simulink model "GA_GearBox"  (R2020a)
settings: Solver=ode23t  StartTime=0.0  StopTime=1  FixedStep=Tsamp  RelTol=1e-3  AbsTol=1e-3  EnableMultiTasking=on
InitFcn:
  | Gear_parameters
StopFcn:
  | Gear_plot
values from neighbouring files (symbols this model uses):
  backlash1_bound = 0.3157*0.1    (= 0.03157)    [Gear_parameters.m]
  backlash2_bound = 0.3157*0.1    (= 0.03157)    [Gear_parameters.m]
  backlash3_bound = 0.2966*0.1    (= 0.02966)    [Gear_parameters.m]
  backlash4_bound = 0.3157*0.1    (= 0.03157)    [Gear_parameters.m]
undefined symbols (not defined in the file or in its folder): sigbuilder_block
libraries: fl_lib x28, nesl_utility x18, sdl_lib x4
Description:
  | Gear with Backlash
settings Model: FPTRunName=Active  ExtModeAutoUpdateStatusClock=off  Creator=MathWorks  LastModifiedBy=JSPark
settings SolverCC: AutoScaleAbsTol=off
settings DataIOCC: MaxDataPoints=10000  SaveFormat=Array  SignalLoggingSaveFormat=ModelDataLogs  SaveOutput=off  SignalLogging=off  DSMLogging=off  ReturnWorkspaceOutputs=off  SignalLoggingName=logsout_sdl_gear_backlash
settings OptimizationCC: ExpressionDepthLimit=2147483647  InitFltsAndDblsToZero=on  LifeSpan=inf
settings DebuggingCC: AlgebraicLoopMsg=none  SaveWithParameterizedLinksMsg=none  SignalResolutionControl=TryResolveAllWithWarning  MultiTaskDSMMsg=warning  MultiTaskCondExecSysMsg=none  SigSpecEnsureSampleTimeMsg=none  StateNameClashWarn=warning  PregeneratedLibrarySubsystemCodeDiagnostic=none  SFUnexpectedBacktrackingDiag=warning  SFNoUnconditionalDefaultTransitionDiag=warning  SFExecutionAtInitializationDiag=none  ArithmeticOperatorsInVariantConditions=warning
settings HardwareCC: ProdBitPerPointer=32  ProdBitPerSizeT=32  ProdBitPerPtrDiffT=32  ProdLargestAtomicFloat=None  ProdIntDivRoundTo=Undefined  ProdEndianess=Unspecified  ProdWordSize=32  ProdHWDeviceType=32-bit Generic  TargetBitPerPointer=64  TargetBitPerSizeT=64  TargetBitPerPtrDiffT=64  TargetLongLongMode=on  TargetIntDivRoundTo=Zero  TargetEndianess=LittleEndian  TargetWordSize=64  TargetHWDeviceType=MATLAB Host  ProdEqTarget=off
settings ModelReferenceCC: PropagateSignalLabelsOutOfModel=off
settings SFSimCC: SimUseLocalCustomCode=off  CustomCodeUndefinedFunction=UseInterfaceOnly
settings RTWCC: Description=Generic Real-Time Target  RTWUseLocalCustomCode=off
settings CodeAppCC: StateflowObjectComments=on
settings GRTTargetCC: TargetLangStandard=C89/C90 (ANSI)  CombineOutputUpdateFcns=off  GRTInterface=on
settings ConfigComp: CovMetricSettings=dw  CovHtmlReporting=on  CovSaveCumulativeToWorkspaceVar=on  CovSaveSingleToWorkspaceVar=on  CovShowResultsExplorer=off  CovExternalEMLEnable=off
settings SimscapeCC: SimscapeLogType=all  SimscapeLogSimulationStatistics=on  SimscapeLogName=simlog_sdl_gear_backlash  SimscapeLogLimitData=off  SimscapeLogDataHistory=15000

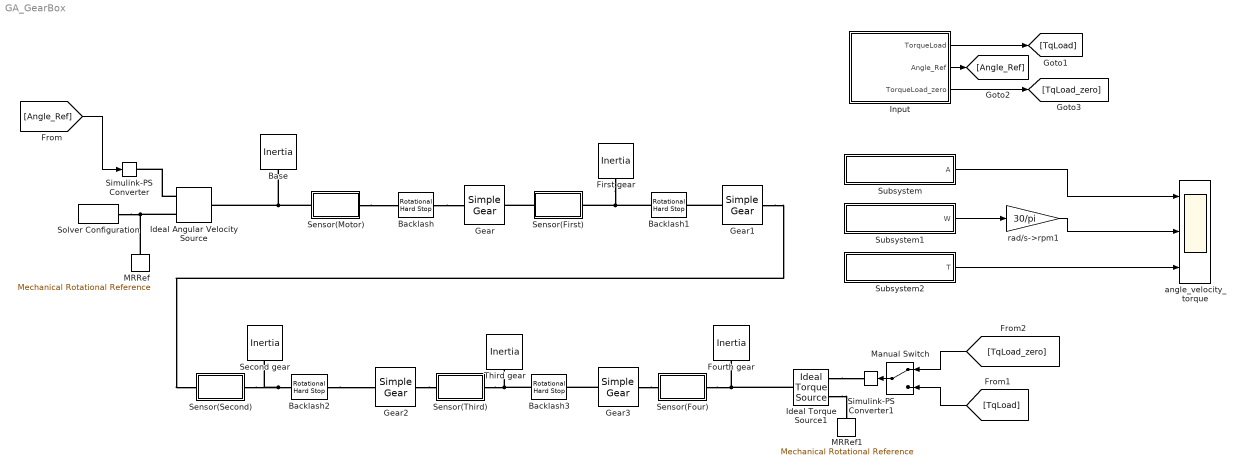
== system GA_GearBox ==
  Backlash : fl_lib/Mechanical/Rotational Elements/Rotational Hard Stop  upper_bnd=backlash1_bound deg  lower_bnd=-backlash1_bound deg  stiff_up=backlash1_stiffness N*m/rad  stiff_low=backlash1_stiffness N*m/rad  D_up=backlash1_damping N*m/(rad/s)  D_low=backlash1_damping N*m/(rad/s)  model=simscape.enum.hardstop.smooth  transition=backlash1_bound*0.1 deg  w_specify=off  w_priority=None  w=0 rad/s  w_nominal_specify=off  w_nominal_unit=rad/s  w_nominal_value=1  t_specify=off  t_priority=None  t=0 N*m  t_nominal_specify=off  t_nominal_unit=N*m  t_nominal_value=1  phi_specify=on  phi_priority=High  phi=0 rad  phi_nominal_specify=off  phi_nominal_unit=rad  phi_nominal_value=1
      settings: SourceProductBaseCode=SS
  Backlash1 : fl_lib/Mechanical/Rotational Elements/Rotational Hard Stop  upper_bnd=backlash2_bound deg  lower_bnd=-backlash2_bound deg  stiff_up=backlash2_stiffness N*m/rad  stiff_low=backlash2_stiffness N*m/rad  D_up=backlash2_damping N*m/(rad/s)  D_low=backlash2_damping N*m/(rad/s)  model=simscape.enum.hardstop.smooth  transition=backlash2_bound*0.1 deg  w_specify=off  w_priority=None  w=0 rad/s  w_nominal_specify=off  w_nominal_unit=rad/s  w_nominal_value=1  t_specify=off  t_priority=None  t=0 N*m  t_nominal_specify=off  t_nominal_unit=N*m  t_nominal_value=1  phi_specify=on  phi_priority=High  phi=0 rad  phi_nominal_specify=off  phi_nominal_unit=rad  phi_nominal_value=1
      settings: SourceProductBaseCode=SS
  Backlash2 : fl_lib/Mechanical/Rotational Elements/Rotational Hard Stop  upper_bnd=backlash3_bound deg  lower_bnd=-backlash3_bound deg  stiff_up=backlash3_stiffness N*m/rad  stiff_low=backlash3_stiffness N*m/rad  D_up=backlash3_damping N*m/(rad/s)  D_low=backlash3_damping N*m/(rad/s)  model=simscape.enum.hardstop.smooth  transition=backlash3_bound*0.1 deg  w_specify=off  w_priority=None  w=0 rad/s  w_nominal_specify=off  w_nominal_unit=rad/s  w_nominal_value=1  t_specify=off  t_priority=None  t=0 N*m  t_nominal_specify=off  t_nominal_unit=N*m  t_nominal_value=1  phi_specify=on  phi_priority=High  phi=0 rad  phi_nominal_specify=off  phi_nominal_unit=rad  phi_nominal_value=1
      settings: SourceProductBaseCode=SS
  Backlash3 : fl_lib/Mechanical/Rotational Elements/Rotational Hard Stop  upper_bnd=backlash4_bound deg  lower_bnd=-backlash4_bound deg  stiff_up=backlash4_stiffness N*m/rad  stiff_low=backlash4_stiffness N*m/rad  D_up=backlash4_damping N*m/(rad/s)  D_low=backlash4_damping N*m/(rad/s)  model=simscape.enum.hardstop.smooth  transition=backlash4_bound*0.1 deg  w_specify=off  w_priority=None  w=0 rad/s  w_nominal_specify=off  w_nominal_unit=rad/s  w_nominal_value=1  t_specify=off  t_priority=None  t=0 N*m  t_nominal_specify=off  t_nominal_unit=N*m  t_nominal_value=1  phi_specify=on  phi_priority=High  phi=0 rad  phi_nominal_specify=off  phi_nominal_unit=rad  phi_nominal_value=1
      settings: SourceProductBaseCode=SS
  Base : fl_lib/Mechanical/Rotational Elements/Inertia  inertia=Jm kg*m^2  w_specify=on  w_priority=High  w=0 rad/s  w_nominal_specify=off  w_nominal_unit=rad/s  w_nominal_value=1  t_specify=off  t_priority=None  t=0 N*m  t_nominal_specify=off  t_nominal_unit=N*m  t_nominal_value=1
  First gear : fl_lib/Mechanical/Rotational Elements/Inertia  inertia=gear_inertia1 kg*m^2  w_specify=on  w_priority=High  w=0 rad/s  w_nominal_specify=off  w_nominal_unit=rad/s  w_nominal_value=1  t_specify=off  t_priority=None  t=0 N*m  t_nominal_specify=off  t_nominal_unit=N*m  t_nominal_value=1
  Fourth gear : fl_lib/Mechanical/Rotational Elements/Inertia  inertia=gear_inertia4 kg*m^2  w_specify=on  w_priority=High  w=0 rad/s  w_nominal_specify=off  w_nominal_unit=rad/s  w_nominal_value=1  t_specify=off  t_priority=None  t=0 N*m  t_nominal_specify=off  t_nominal_unit=N*m  t_nominal_value=1
  Gear : sdl_lib/Gears/Simple Gear  ratio=gear_ratio1  rotation_direction=1  friction_model=sdl.enum.gear_efficiencies_load.off  T_noload=0.1 N*m  T_nom=5 N*m  efficiency_nom=0.8  efficiency=0.8  mu_visc=[ 0 0 ] N*m/(rad/s)  w_thr=0.01 rad/s  pwr_thr=0.001 W  enable_faults=simscape.enum.onoff.off  efficiency_fault=0.05  external_fault=simscape.enum.onoff.off  temporal_fault=simscape.enum.onoff.off  fault_time=5 s  fault_angles=pi / 12 rad  report_fault=1  temperature_TLU=[ 280 300 320 ] K  load_TLU=[ 1 5 10 ] N*m  efficiency_TLU=[ 0.95 0.9 0.85 ]  efficiency_TLU2=[ 0.85 0.8 0.75; 0.95 0.9 0.85; 0.85 0.8 0.7 ]  thermal_mass=50 J/K  T_init=300 K
  Gear1 : sdl_lib/Gears/Simple Gear  ratio=gear_ratio2  rotation_direction=1  friction_model=sdl.enum.gear_efficiencies_load.off  T_noload=0.1 N*m  T_nom=5 N*m  efficiency_nom=0.8  efficiency=0.8  mu_visc=[ 0 0 ] N*m/(rad/s)  w_thr=0.01 rad/s  pwr_thr=0.001 W  enable_faults=simscape.enum.onoff.off  efficiency_fault=0.05  external_fault=simscape.enum.onoff.off  temporal_fault=simscape.enum.onoff.off  fault_time=5 s  fault_angles=pi / 12 rad  report_fault=1  temperature_TLU=[ 280 300 320 ] K  load_TLU=[ 1 5 10 ] N*m  efficiency_TLU=[ 0.95 0.9 0.85 ]  efficiency_TLU2=[ 0.85 0.8 0.75; 0.95 0.9 0.85; 0.85 0.8 0.7 ]  thermal_mass=50 J/K  T_init=300 K
  Gear2 : sdl_lib/Gears/Simple Gear  ratio=gear_ratio3  rotation_direction=1  friction_model=sdl.enum.gear_efficiencies_load.off  T_noload=0.1 N*m  T_nom=5 N*m  efficiency_nom=0.8  efficiency=0.8  mu_visc=[ 0 0 ] N*m/(rad/s)  w_thr=0.01 rad/s  pwr_thr=0.001 W  enable_faults=simscape.enum.onoff.off  efficiency_fault=0.05  external_fault=simscape.enum.onoff.off  temporal_fault=simscape.enum.onoff.off  fault_time=5 s  fault_angles=pi / 12 rad  report_fault=1  temperature_TLU=[ 280 300 320 ] K  load_TLU=[ 1 5 10 ] N*m  efficiency_TLU=[ 0.95 0.9 0.85 ]  efficiency_TLU2=[ 0.85 0.8 0.75; 0.95 0.9 0.85; 0.85 0.8 0.7 ]  thermal_mass=50 J/K  T_init=300 K
  Gear3 : sdl_lib/Gears/Simple Gear  ratio=gear_ratio4  rotation_direction=1  friction_model=sdl.enum.gear_efficiencies_load.off  T_noload=0.1 N*m  T_nom=5 N*m  efficiency_nom=0.8  efficiency=0.8  mu_visc=[ 0 0 ] N*m/(rad/s)  w_thr=0.01 rad/s  pwr_thr=0.001 W  enable_faults=simscape.enum.onoff.off  efficiency_fault=0.05  external_fault=simscape.enum.onoff.off  temporal_fault=simscape.enum.onoff.off  fault_time=5 s  fault_angles=pi / 12 rad  report_fault=1  temperature_TLU=[ 280 300 320 ] K  load_TLU=[ 1 5 10 ] N*m  efficiency_TLU=[ 0.95 0.9 0.85 ]  efficiency_TLU2=[ 0.85 0.8 0.75; 0.95 0.9 0.85; 0.85 0.8 0.7 ]  thermal_mass=50 J/K  T_init=300 K
  Ideal Angular Velocity Source : fl_lib/Mechanical/Mechanical Sources/Ideal Angular Velocity Source
  Ideal Torque Source1 : fl_lib/Mechanical/Mechanical Sources/Ideal Torque Source
  Input : Subsystem  Tag=STV Subsys  LoadFcn=sigbuilder_block('load');  StartFcn=sigbuilder_block('start');  StopFcn=sigbuilder_block('stop');  ClipboardFcn=sigbuilder_block('clipboard');  mask(Sigbuilder block){tuvar=[0:10]}
      mask help: Simulink:masks:SigbuilderBlock_MD
      mask init:
      | if ~strcmp(get_param(bdroot(gcbh),'SimulationStatus'),'stopped') tuvar = sigbuilder_block('maskInit'); end
      settings: CopyFcn=sigbuilder_block('copy');  DeleteFcn=sigbuilder_block('delete');  ModelCloseFcn=sigbuilder_block('modelClose');  PreSaveFcn=sigbuilder_block('preSave');  PauseFcn=sigbuilder_block('pause');  ContinueFcn=sigbuilder_block('continue');  NameChangeFcn=sigbuilder_block('namechange');  OpenFcn=sigbuilder_block('open',[661.5 288 949.5 474.75 ]);  CloseFcn=sigbuilder_block('close');
      mask Display: plot(0, 0, 100, 100,[2, 2, 32, 32, 2], [68, 8, 8, 68, 68],[32, 2], [38, 38], [32, 19, 2],[53, 60, 44], [32, 17, 17, 2],[16, 16, 31, 31]);txt = getActiveGroup(gcbh);text(2, 100, txt,'verticalAlignment', 'top');
  MRRef : fl_lib/Mechanical/Rotational Elements/Mechanical Rotational Reference
  MRRef1 : fl_lib/Mechanical/Rotational Elements/Mechanical Rotational Reference
  Manual Switch : ManualSwitch
  Second gear : fl_lib/Mechanical/Rotational Elements/Inertia  inertia=gear_inertia2 kg*m^2  w_specify=on  w_priority=High  w=0 rad/s  w_nominal_specify=off  w_nominal_unit=rad/s  w_nominal_value=1  t_specify=off  t_priority=None  t=0 N*m  t_nominal_specify=off  t_nominal_unit=N*m  t_nominal_value=1
  Sensor(First) : Subsystem
  Sensor(Four) : Subsystem
  Sensor(Motor) : Subsystem
  Sensor(Second) : Subsystem
  Sensor(Third) : Subsystem
  Simulink-PS Converter : nesl_utility/Simulink-PS Converter  PhysicalDomain=network_engine_domain  SubClassName=ps_input  LeftPortType=input  RightPortType=output  PseudoPeriodic=off  Frequencies=[]  NoiseDistribution=none  NoiseParameters=[]  Unit=1  AffineConversion=off  FilteringAndDerivatives=filter  SimscapeFilterOrder=1  InputFilterTimeConstant=0.001  UdotUserProvided=0
  Simulink-PS Converter1 : nesl_utility/Simulink-PS Converter  PhysicalDomain=network_engine_domain  SubClassName=ps_input  LeftPortType=input  RightPortType=output  PseudoPeriodic=off  Frequencies=[]  NoiseDistribution=none  NoiseParameters=[]  Unit=1  AffineConversion=off  FilteringAndDerivatives=provide  SimscapeFilterOrder=1  InputFilterTimeConstant=0.001  UdotUserProvided=0
  Solver Configuration : nesl_utility/Solver Configuration  PhysicalDomain=network_engine_domain  SubClassName=solver  LeftPortType=input  RightPortType=generic  Tones=[]  Harmonics=[]  SimulateNoise=off  Profile=off  UseLocalSampling=off  EnableSwitchedLinearOptims=on  FrequencyDomain=off  UseCCode=off  RelTol=0.001  AbsTol=1e-06  MinStep=1e-09  ToWorkspace=off  RevertToSquareIcSolve=off  NumHomotopyIterations=100  PhasorMode=off  PhasorModeNumHarmonics=1  DoDC=off  ResidualTolerance=1e-9  UseLocalSolver=off  LocalSolverChoice=NE_PARTITIONING_ADVANCER  LocalSolverSampleTime=0.0001  DoFixedCost=off  MaxNonlinIter=3  MaxModeIter=2  LinearAlgebra=auto  EquationFormulation=NE_TIME_EF  DelaysMemoryBudget=1024  AutomaticFiltering=on  FilteringTimeConstant=0.001  PartitionStorageMethod=EXHAUSTIVE  PartitionMemoryBudget=1024  PartitionMethod=ROBUST
  Subsystem : Subsystem
  Subsystem1 : Subsystem
  Subsystem2 : Subsystem
  Third gear : fl_lib/Mechanical/Rotational Elements/Inertia  inertia=gear_inertai3 kg*m^2  w_specify=on  w_priority=High  w=0 rad/s  w_nominal_specify=off  w_nominal_unit=rad/s  w_nominal_value=1  t_specify=off  t_priority=None  t=0 N*m  t_nominal_specify=off  t_nominal_unit=N*m  t_nominal_value=1
  angle_velocity_torque : Scope  NumInputPorts=3
      settings: Tag=angle,velocity,torque  Description=angle,velocity,torque
  rad/s->rpm1 : Gain  Gain=30/pi
  wires:
  Subsystem2/1(T) -> angle_velocity_torque/3
  Input/1(TorqueLoad) -> [TqLoad]
  Subsystem/1(A) -> angle_velocity_torque/1
  Input/2(Angle_Ref) -> [Angle_Ref]
  Subsystem1/1(W) -> rad/s->rpm1/1
  [Angle_Ref] -> Simulink-PS Converter/1
  rad/s->rpm1/1 -> angle_velocity_torque/2
  Input/3(TorqueLoad_zero) -> [TqLoad_zero]
  Manual Switch/1 -> Simulink-PS Converter1/1
  [TqLoad] -> Manual Switch/2
  [TqLoad_zero] -> Manual Switch/1
  connections:
  Sensor(Four)/RConn1 -- Ideal Torque Source1/LConn1 -- Fourth gear/LConn1
  Backlash2/LConn1 -- Second gear/LConn1 -- Sensor(Second)/RConn1
  MRRef/LConn1 -- Ideal Angular Velocity Source/RConn2 -- Solver Configuration/RConn1
  Sensor(Motor)/LConn1 -- Ideal Angular Velocity Source/LConn1 -- Base/LConn1
  First gear/LConn1 -- Sensor(First)/RConn1 -- Backlash1/LConn1
  Backlash3/LConn1 -- Sensor(Third)/RConn1 -- Third gear/LConn1
  Ideal Torque Source1/RConn1 -- Simulink-PS Converter1/RConn1
  Sensor(First)/LConn1 -- Gear/RConn1
  Backlash2/RConn1 -- Gear2/LConn1
  Ideal Angular Velocity Source/RConn1 -- Simulink-PS Converter/RConn1
  Sensor(Motor)/RConn1 -- Backlash/LConn1
  Gear2/RConn1 -- Sensor(Third)/LConn1
  Backlash/RConn1 -- Gear/LConn1
  Gear3/RConn1 -- Sensor(Four)/LConn1
  Gear1/LConn1 -- Backlash1/RConn1
  Gear3/LConn1 -- Backlash3/RConn1
  Gear1/RConn1 -- Sensor(Second)/LConn1
  Ideal Torque Source1/RConn2 -- MRRef1/LConn1

== system GA_GearBox/Input ==
  Demux : Demux  Tag=STV Demux  Outputs=3
      settings: DisplayOption=none
  FromWs : FromWorkspace  Tag=STV FromWs  VariableName=tuvar
      SigBuilderData=|
      | common.afterFinalStr = 'Extrapolate'
      | common.sampleTime = 0
      | dataSet.timeRange = [0 1]
      | dataSet.name = 'Test 1'
      | sbobj.Groups.Name = 'Test 1'
      | sbobj.Groups.Signals(1).Name = 'TorqueLoad'
      | sbobj.Groups.Signals(1).XData = [0 0.1 0.4 0.5 0.6 0.9 1]
      | sbobj.Groups.Signals(1).YData = [0 50 50 0 -50 -50 0]
      | sbobj.Groups.Signals(2).Name = 'Angle_Ref'
      | sbobj.Groups.Signals(2).XData = [0 0.2 0.6 1]
      | sbobj.Groups.Signals(2).YData = [0 0 418.88 418.88]
      | sbobj.Groups.Signals(3).Name = 'TorqueLoad_zero'
      | sbobj.Groups.Signals(3).XData = [0 1]
      | sbobj.Groups.Signals(3).YData = [0 0]
      | sbobj.Groups.TimeRange = [0 1]
  TorqueLoad : Outport  Tag=STV Outport  VectorParamsAs1DForOutWhenUnconnected=off
  Angle_Ref : Outport  Tag=STV Outport  Port=2  VectorParamsAs1DForOutWhenUnconnected=off
  TorqueLoad_zero : Outport  Tag=STV Outport  Port=3
  wires:
  Demux/1 -> TorqueLoad/1
  FromWs/1 -> Demux/1
  Demux/2 -> Angle_Ref/1
  Demux/3 -> TorqueLoad_zero/1

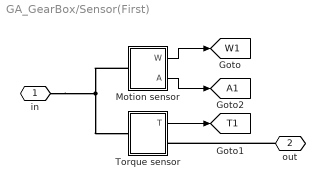
== system GA_GearBox/Sensor(First) ==
  Motion sensor : Subsystem
  Torque sensor : Subsystem
  in : PMIOPort  Side=Left
  out : PMIOPort  Port=2  Side=Right
  tag scope: A1=global, T1=global, W1=global
  wires:
  Motion sensor/1(W) -> [W1]
  Torque sensor/1(T) -> [T1]
  Motion sensor/2(A) -> [A1]
  connections:
  in/RConn1 -- Motion sensor/LConn1 -- Torque sensor/LConn1
  out/RConn1 -- Torque sensor/RConn1

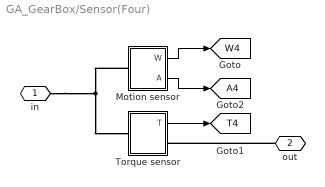
== system GA_GearBox/Sensor(Four) ==
  Motion sensor : Subsystem
  Torque sensor : Subsystem
  in : PMIOPort  Side=Left
  out : PMIOPort  Port=2  Side=Right
  tag scope: A4=global, T4=global, W4=global
  wires:
  Motion sensor/1(W) -> [W4]
  Torque sensor/1(T) -> [T4]
  Motion sensor/2(A) -> [A4]
  connections:
  in/RConn1 -- Motion sensor/LConn1 -- Torque sensor/LConn1
  out/RConn1 -- Torque sensor/RConn1

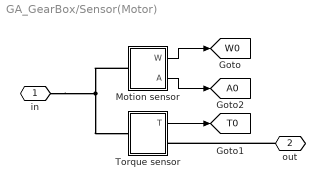
== system GA_GearBox/Sensor(Motor) ==
  Motion sensor : Subsystem
  Torque sensor : Subsystem
  in : PMIOPort  Side=Left
  out : PMIOPort  Port=2  Side=Right
  tag scope: A0=global, T0=global, W0=global
  wires:
  Motion sensor/1(W) -> [W0]
  Torque sensor/1(T) -> [T0]
  Motion sensor/2(A) -> [A0]
  connections:
  in/RConn1 -- Motion sensor/LConn1 -- Torque sensor/LConn1
  out/RConn1 -- Torque sensor/RConn1

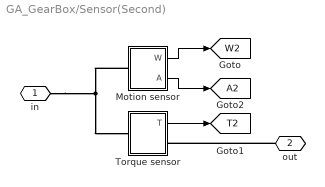
== system GA_GearBox/Sensor(Second) ==
  Motion sensor : Subsystem
  Torque sensor : Subsystem
  in : PMIOPort  Side=Left
  out : PMIOPort  Port=2  Side=Right
  tag scope: A2=global, T2=global, W2=global
  wires:
  Motion sensor/1(W) -> [W2]
  Torque sensor/1(T) -> [T2]
  Motion sensor/2(A) -> [A2]
  connections:
  in/RConn1 -- Motion sensor/LConn1 -- Torque sensor/LConn1
  out/RConn1 -- Torque sensor/RConn1

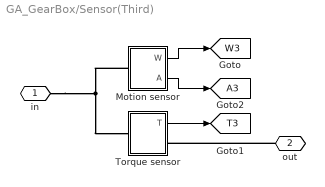
== system GA_GearBox/Sensor(Third) ==
  Motion sensor : Subsystem
  Torque sensor : Subsystem
  in : PMIOPort  Side=Left
  out : PMIOPort  Port=2  Side=Right
  tag scope: A3=global, T3=global, W3=global
  wires:
  Motion sensor/1(W) -> [W3]
  Torque sensor/1(T) -> [T3]
  Motion sensor/2(A) -> [A3]
  connections:
  in/RConn1 -- Motion sensor/LConn1 -- Torque sensor/LConn1
  out/RConn1 -- Torque sensor/RConn1

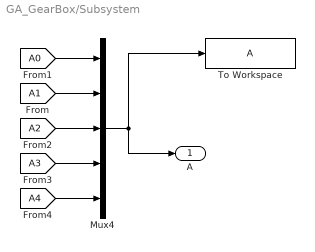
== system GA_GearBox/Subsystem ==
  Mux4 : Mux  Inputs=5
  To Workspace : ToWorkspace  VariableName=A  SaveFormat=Timeseries  SampleTime=-1
  A : Outport
  wires:
  Mux4/1 -> A/1, To Workspace/1
  [A4] -> Mux4/5
  [A3] -> Mux4/4
  [A2] -> Mux4/3
  [A1] -> Mux4/2
  [A0] -> Mux4/1

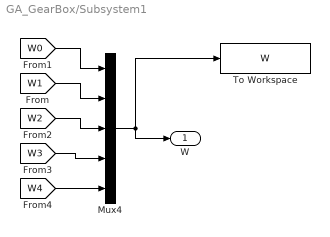
== system GA_GearBox/Subsystem1 ==
  Mux4 : Mux  Inputs=5
  To Workspace : ToWorkspace  VariableName=W  SaveFormat=Timeseries  SampleTime=-1
  W : Outport
  wires:
  Mux4/1 -> W/1, To Workspace/1
  [W4] -> Mux4/5
  [W3] -> Mux4/4
  [W2] -> Mux4/3
  [W1] -> Mux4/2
  [W0] -> Mux4/1

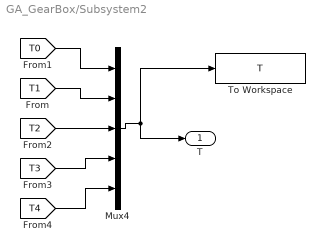
== system GA_GearBox/Subsystem2 ==
  Mux4 : Mux  Inputs=5
  To Workspace : ToWorkspace  VariableName=T  SaveFormat=Timeseries  SampleTime=-1
  T : Outport
  wires:
  Mux4/1 -> T/1, To Workspace/1
  [T0] -> Mux4/1
  [T1] -> Mux4/2
  [T2] -> Mux4/3
  [T3] -> Mux4/4
  [T4] -> Mux4/5

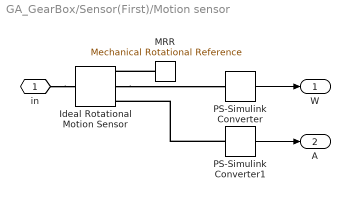
== system GA_GearBox/Sensor(First)/Motion sensor ==
  Ideal Rotational Motion Sensor : fl_lib/Mechanical/Mechanical Sensors/Ideal Rotational Motion Sensor  wrap_angle=simscape.enum.onoff.off  offset=0 rad
  MRR : fl_lib/Mechanical/Rotational Elements/Mechanical Rotational Reference
  PS-Simulink Converter : nesl_utility/PS-Simulink Converter  PhysicalDomain=network_engine_domain  SubClassName=ps_output  LeftPortType=input  RightPortType=output  PseudoPeriodic=off  Frequencies=[]  Unit=rad/s  AffineConversion=off
  PS-Simulink Converter1 : nesl_utility/PS-Simulink Converter  PhysicalDomain=network_engine_domain  SubClassName=ps_output  LeftPortType=input  RightPortType=output  PseudoPeriodic=off  Frequencies=[]  Unit=rad  AffineConversion=off
  in : PMIOPort  Side=Left
  W : Outport  VectorParamsAs1DForOutWhenUnconnected=off
  A : Outport  Port=2  VectorParamsAs1DForOutWhenUnconnected=off
  wires:
  PS-Simulink Converter/1 -> W/1
  PS-Simulink Converter1/1 -> A/1
  connections:
  in/RConn1 -- Ideal Rotational Motion Sensor/LConn1
  Ideal Rotational Motion Sensor/RConn2 -- PS-Simulink Converter/LConn1
  MRR/LConn1 -- Ideal Rotational Motion Sensor/RConn1
  PS-Simulink Converter1/LConn1 -- Ideal Rotational Motion Sensor/RConn3

== system GA_GearBox/Sensor(First)/Torque sensor ==
  PS2S : nesl_utility/PS-Simulink Converter  PhysicalDomain=network_engine_domain  SubClassName=ps_output  LeftPortType=input  RightPortType=output  PseudoPeriodic=off  Frequencies=[]  Unit=N*m  AffineConversion=off
  Torque Sensor : fl_lib/Mechanical/Mechanical Sensors/Ideal Torque Sensor
  B : PMIOPort  Side=Right
  in : PMIOPort  Port=2  Side=Left
  T : Outport  VectorParamsAs1DForOutWhenUnconnected=off
  wires:
  PS2S/1 -> T/1
  connections:
  in/RConn1 -- Torque Sensor/LConn1
  B/RConn1 -- Torque Sensor/RConn1
  Torque Sensor/RConn2 -- PS2S/LConn1

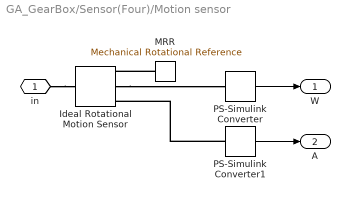
== system GA_GearBox/Sensor(Four)/Motion sensor ==
  Ideal Rotational Motion Sensor : fl_lib/Mechanical/Mechanical Sensors/Ideal Rotational Motion Sensor  wrap_angle=simscape.enum.onoff.off  offset=0 rad
  MRR : fl_lib/Mechanical/Rotational Elements/Mechanical Rotational Reference
  PS-Simulink Converter : nesl_utility/PS-Simulink Converter  PhysicalDomain=network_engine_domain  SubClassName=ps_output  LeftPortType=input  RightPortType=output  PseudoPeriodic=off  Frequencies=[]  Unit=rad/s  AffineConversion=off
  PS-Simulink Converter1 : nesl_utility/PS-Simulink Converter  PhysicalDomain=network_engine_domain  SubClassName=ps_output  LeftPortType=input  RightPortType=output  PseudoPeriodic=off  Frequencies=[]  Unit=rad  AffineConversion=off
  in : PMIOPort  Side=Left
  W : Outport  VectorParamsAs1DForOutWhenUnconnected=off
  A : Outport  Port=2  VectorParamsAs1DForOutWhenUnconnected=off
  wires:
  PS-Simulink Converter/1 -> W/1
  PS-Simulink Converter1/1 -> A/1
  connections:
  in/RConn1 -- Ideal Rotational Motion Sensor/LConn1
  Ideal Rotational Motion Sensor/RConn2 -- PS-Simulink Converter/LConn1
  MRR/LConn1 -- Ideal Rotational Motion Sensor/RConn1
  PS-Simulink Converter1/LConn1 -- Ideal Rotational Motion Sensor/RConn3

== system GA_GearBox/Sensor(Four)/Torque sensor ==
  PS2S : nesl_utility/PS-Simulink Converter  PhysicalDomain=network_engine_domain  SubClassName=ps_output  LeftPortType=input  RightPortType=output  PseudoPeriodic=off  Frequencies=[]  Unit=N*m  AffineConversion=off
  Torque Sensor : fl_lib/Mechanical/Mechanical Sensors/Ideal Torque Sensor
  B : PMIOPort  Side=Right
  in : PMIOPort  Port=2  Side=Left
  T : Outport  VectorParamsAs1DForOutWhenUnconnected=off
  wires:
  PS2S/1 -> T/1
  connections:
  in/RConn1 -- Torque Sensor/LConn1
  B/RConn1 -- Torque Sensor/RConn1
  Torque Sensor/RConn2 -- PS2S/LConn1

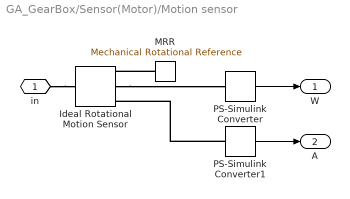
== system GA_GearBox/Sensor(Motor)/Motion sensor ==
  Ideal Rotational Motion Sensor : fl_lib/Mechanical/Mechanical Sensors/Ideal Rotational Motion Sensor  wrap_angle=simscape.enum.onoff.off  offset=0 rad
  MRR : fl_lib/Mechanical/Rotational Elements/Mechanical Rotational Reference
  PS-Simulink Converter : nesl_utility/PS-Simulink Converter  PhysicalDomain=network_engine_domain  SubClassName=ps_output  LeftPortType=input  RightPortType=output  PseudoPeriodic=off  Frequencies=[]  Unit=rad/s  AffineConversion=off
  PS-Simulink Converter1 : nesl_utility/PS-Simulink Converter  PhysicalDomain=network_engine_domain  SubClassName=ps_output  LeftPortType=input  RightPortType=output  PseudoPeriodic=off  Frequencies=[]  Unit=rad  AffineConversion=off
  in : PMIOPort  Side=Left
  W : Outport  VectorParamsAs1DForOutWhenUnconnected=off
  A : Outport  Port=2  VectorParamsAs1DForOutWhenUnconnected=off
  wires:
  PS-Simulink Converter/1 -> W/1
  PS-Simulink Converter1/1 -> A/1
  connections:
  in/RConn1 -- Ideal Rotational Motion Sensor/LConn1
  Ideal Rotational Motion Sensor/RConn2 -- PS-Simulink Converter/LConn1
  MRR/LConn1 -- Ideal Rotational Motion Sensor/RConn1
  PS-Simulink Converter1/LConn1 -- Ideal Rotational Motion Sensor/RConn3

== system GA_GearBox/Sensor(Motor)/Torque sensor ==
  PS2S : nesl_utility/PS-Simulink Converter  PhysicalDomain=network_engine_domain  SubClassName=ps_output  LeftPortType=input  RightPortType=output  PseudoPeriodic=off  Frequencies=[]  Unit=N*m  AffineConversion=off
  Torque Sensor : fl_lib/Mechanical/Mechanical Sensors/Ideal Torque Sensor
  B : PMIOPort  Side=Right
  in : PMIOPort  Port=2  Side=Left
  T : Outport  VectorParamsAs1DForOutWhenUnconnected=off
  wires:
  PS2S/1 -> T/1
  connections:
  in/RConn1 -- Torque Sensor/LConn1
  B/RConn1 -- Torque Sensor/RConn1
  Torque Sensor/RConn2 -- PS2S/LConn1

== system GA_GearBox/Sensor(Second)/Motion sensor ==
  Ideal Rotational Motion Sensor : fl_lib/Mechanical/Mechanical Sensors/Ideal Rotational Motion Sensor  wrap_angle=simscape.enum.onoff.off  offset=0 rad
  MRR : fl_lib/Mechanical/Rotational Elements/Mechanical Rotational Reference
  PS-Simulink Converter : nesl_utility/PS-Simulink Converter  PhysicalDomain=network_engine_domain  SubClassName=ps_output  LeftPortType=input  RightPortType=output  PseudoPeriodic=off  Frequencies=[]  Unit=rad/s  AffineConversion=off
  PS-Simulink Converter1 : nesl_utility/PS-Simulink Converter  PhysicalDomain=network_engine_domain  SubClassName=ps_output  LeftPortType=input  RightPortType=output  PseudoPeriodic=off  Frequencies=[]  Unit=rad  AffineConversion=off
  in : PMIOPort  Side=Left
  W : Outport  VectorParamsAs1DForOutWhenUnconnected=off
  A : Outport  Port=2  VectorParamsAs1DForOutWhenUnconnected=off
  wires:
  PS-Simulink Converter/1 -> W/1
  PS-Simulink Converter1/1 -> A/1
  connections:
  in/RConn1 -- Ideal Rotational Motion Sensor/LConn1
  Ideal Rotational Motion Sensor/RConn2 -- PS-Simulink Converter/LConn1
  MRR/LConn1 -- Ideal Rotational Motion Sensor/RConn1
  PS-Simulink Converter1/LConn1 -- Ideal Rotational Motion Sensor/RConn3

== system GA_GearBox/Sensor(Second)/Torque sensor ==
  PS2S : nesl_utility/PS-Simulink Converter  PhysicalDomain=network_engine_domain  SubClassName=ps_output  LeftPortType=input  RightPortType=output  PseudoPeriodic=off  Frequencies=[]  Unit=N*m  AffineConversion=off
  Torque Sensor : fl_lib/Mechanical/Mechanical Sensors/Ideal Torque Sensor
  B : PMIOPort  Side=Right
  in : PMIOPort  Port=2  Side=Left
  T : Outport  VectorParamsAs1DForOutWhenUnconnected=off
  wires:
  PS2S/1 -> T/1
  connections:
  in/RConn1 -- Torque Sensor/LConn1
  B/RConn1 -- Torque Sensor/RConn1
  Torque Sensor/RConn2 -- PS2S/LConn1

== system GA_GearBox/Sensor(Third)/Motion sensor ==
  Ideal Rotational Motion Sensor : fl_lib/Mechanical/Mechanical Sensors/Ideal Rotational Motion Sensor  wrap_angle=simscape.enum.onoff.off  offset=0 rad
  MRR : fl_lib/Mechanical/Rotational Elements/Mechanical Rotational Reference
  PS-Simulink Converter : nesl_utility/PS-Simulink Converter  PhysicalDomain=network_engine_domain  SubClassName=ps_output  LeftPortType=input  RightPortType=output  PseudoPeriodic=off  Frequencies=[]  Unit=rad/s  AffineConversion=off
  PS-Simulink Converter1 : nesl_utility/PS-Simulink Converter  PhysicalDomain=network_engine_domain  SubClassName=ps_output  LeftPortType=input  RightPortType=output  PseudoPeriodic=off  Frequencies=[]  Unit=rad  AffineConversion=off
  in : PMIOPort  Side=Left
  W : Outport  VectorParamsAs1DForOutWhenUnconnected=off
  A : Outport  Port=2  VectorParamsAs1DForOutWhenUnconnected=off
  wires:
  PS-Simulink Converter/1 -> W/1
  PS-Simulink Converter1/1 -> A/1
  connections:
  in/RConn1 -- Ideal Rotational Motion Sensor/LConn1
  Ideal Rotational Motion Sensor/RConn2 -- PS-Simulink Converter/LConn1
  MRR/LConn1 -- Ideal Rotational Motion Sensor/RConn1
  PS-Simulink Converter1/LConn1 -- Ideal Rotational Motion Sensor/RConn3

== system GA_GearBox/Sensor(Third)/Torque sensor ==
  PS2S : nesl_utility/PS-Simulink Converter  PhysicalDomain=network_engine_domain  SubClassName=ps_output  LeftPortType=input  RightPortType=output  PseudoPeriodic=off  Frequencies=[]  Unit=N*m  AffineConversion=off
  Torque Sensor : fl_lib/Mechanical/Mechanical Sensors/Ideal Torque Sensor
  B : PMIOPort  Side=Right
  in : PMIOPort  Port=2  Side=Left
  T : Outport  VectorParamsAs1DForOutWhenUnconnected=off
  wires:
  PS2S/1 -> T/1
  connections:
  in/RConn1 -- Torque Sensor/LConn1
  B/RConn1 -- Torque Sensor/RConn1
  Torque Sensor/RConn2 -- PS2S/LConn1
